simulink model "LAB_6_part2"  (R2015a)
settings: Solver=ode45  StartTime=0.0  StopTime=10.0  RelTol=1e-3
libraries: arduinolib x2, simulink x1, RASPlib x1
settings Model: Creator=009891752  LastModifiedBy=009891752

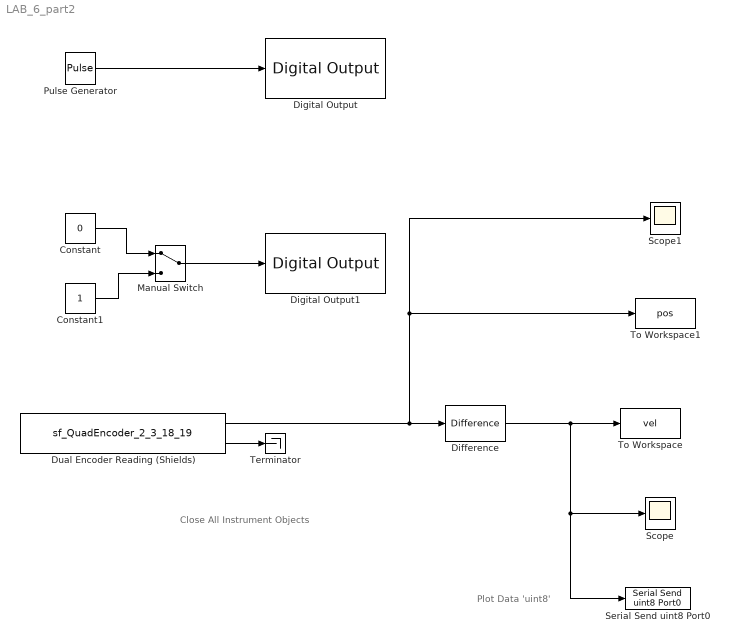
== system LAB_6_part2 ==
  note: Plot Data
      | 'uint8'
  note: Close All
      | Instrument Objects
  Constant : Constant  Value=0
  Constant1 : Constant
  Difference : simulink/Discrete/Difference  ICPrevInput=0.0  InputProcessing=Inherited  OutMin=[]  OutMax=[]  OutDataType=fixdt(1, 16)  OutScaling=2^-10  DoSatur=off
  Digital Output : arduinolib/Digital Output  pinNumber=9  blockPlatform=arduino
  Digital Output1 : arduinolib/Digital Output  pinNumber=5  blockPlatform=arduino
  Dual Encoder Reading (Shields) : S-Function  InitFcn=try, set_param(gcb,'FunctionName','sf_QuadEncoder_2_3_18_19'), end  FunctionName=sf_QuadEncoder_2_3_18_19  Parameters=uint8([0 1]),uint8([2 18]),uint8([3 19])  SFunctionModules=sf_QuadEncoder_2_3_18_19_wrapper  mask(S-Function Builder){}
      mask init:
      | val = [[.9  0.75 0.75 1 1 .9 .9 1]',[1 1 0.75 0.75 .9 .9 1 .9]'];try , sys = get_param(gcb,'SfunBuilderFcnName');if isempty(sys), sys = get_param(gcb,'FunctionName'); end,catch, sys = get_param(gcb,'FunctionName'); end
      settings: CopyFcn=set_param(gcbh,'LinkStatus','none')  PreSaveFcn=try, set_param(gcb,'FunctionName','sf_QuadEncoder_2_3_18_19'), end  OpenFcn=sfunctionwizard(gcbh)
      mask Display: plot(val(:,1),val(:,2)),disp(sys), port_label('output',1,'pos1'), port_label('output',2,'pos2')
  Manual Switch : ManualSwitch
  Pulse Generator : DiscretePulseGenerator  PulseType=Time based  Period=10  PulseWidth=5
  Scope : Scope
  Scope1 : Scope
  Serial Send uint8 Port0 : RASPlib/Serial Send uint8 Port0
  Terminator : Terminator
  To Workspace : ToWorkspace  VariableName=vel  SaveFormat=Timeseries  SampleTime=-1
  To Workspace1 : ToWorkspace  VariableName=pos  SaveFormat=Timeseries  SampleTime=-1
  wires:
  Pulse Generator/1 -> Digital Output/1
  Constant/1 -> Manual Switch/1
  Constant1/1 -> Manual Switch/2
  Manual Switch/1 -> Digital Output1/1
  Dual Encoder Reading (Shields)/2 -> Terminator/1
  Dual Encoder Reading (Shields)/1 -> To Workspace1/1, Scope1/1, Difference/1
  Difference/1 -> Serial Send uint8 Port0/1, Scope/1, To Workspace/1
